simulink model "TST_AirCtl_DesValCalc"  (R2016b)
settings: Solver=FixedStepDiscrete  StartTime=0.0  StopTime=simTime  FixedStep=sampleTime  RelTol=1e-3
values from neighbouring files (symbols this model uses):
  testCase = 1    [initTST_AirCtl_DesValCalc_001.m]
libraries: simulink x4, UnitTest_Lib x2
settings Model: Creator=zhulinfeng  LastModifiedBy=zhulinfeng
settings DebuggingCC: SignalRangeChecking=error

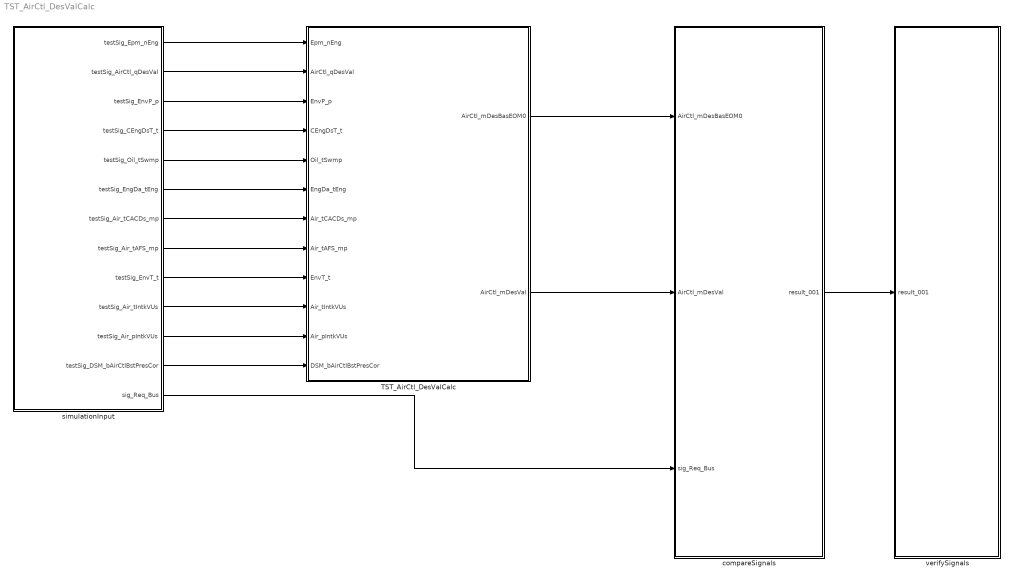
== system TST_AirCtl_DesValCalc ==
  TST_AirCtl_DesValCalc : Subsystem
  compareSignals : Subsystem
  simulationInput : Subsystem
  verifySignals : Subsystem
  wires:
  simulationInput/1(testSig_Epm_nEng) -> TST_AirCtl_DesValCalc/1(Epm_nEng)
  simulationInput/2(testSig_AirCtl_qDesVal) -> TST_AirCtl_DesValCalc/2(AirCtl_qDesVal)
  simulationInput/3(testSig_EnvP_p) -> TST_AirCtl_DesValCalc/3(EnvP_p)
  simulationInput/4(testSig_CEngDsT_t) -> TST_AirCtl_DesValCalc/4(CEngDsT_t)
  simulationInput/5(testSig_Oil_tSwmp) -> TST_AirCtl_DesValCalc/5(Oil_tSwmp)
  simulationInput/6(testSig_EngDa_tEng) -> TST_AirCtl_DesValCalc/6(EngDa_tEng)
  simulationInput/7(testSig_Air_tCACDs_mp) -> TST_AirCtl_DesValCalc/7(Air_tCACDs_mp)
  simulationInput/8(testSig_Air_tAFS_mp) -> TST_AirCtl_DesValCalc/8(Air_tAFS_mp)
  simulationInput/9(testSig_EnvT_t) -> TST_AirCtl_DesValCalc/9(EnvT_t)
  simulationInput/10(testSig_Air_tIntkVUs) -> TST_AirCtl_DesValCalc/10(Air_tIntkVUs)
  simulationInput/11(testSig_Air_pIntkVUs) -> TST_AirCtl_DesValCalc/11(Air_pIntkVUs)
  simulationInput/12(testSig_DSM_bAirCtlBstPresCor) -> TST_AirCtl_DesValCalc/12(DSM_bAirCtlBstPresCor)
  TST_AirCtl_DesValCalc/1(AirCtl_mDesBasEOM0) -> compareSignals/1(AirCtl_mDesBasEOM0)
  TST_AirCtl_DesValCalc/2(AirCtl_mDesVal) -> compareSignals/2(AirCtl_mDesVal)
  simulationInput/13(sig_Req_Bus) -> compareSignals/3(sig_Req_Bus)
  compareSignals/1(result_001) -> verifySignals/1(result_001)

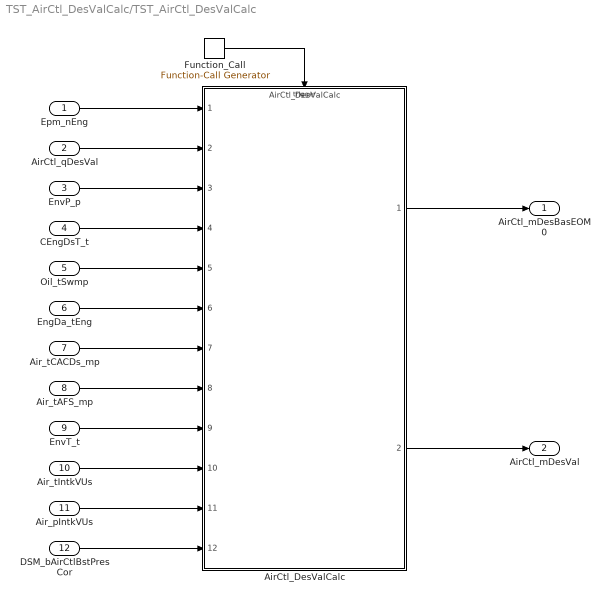
== system TST_AirCtl_DesValCalc/TST_AirCtl_DesValCalc ==
  Epm_nEng : Inport
  AirCtl_qDesVal : Inport  Port=2
  EnvP_p : Inport  Port=3
  CEngDsT_t : Inport  Port=4
  Oil_tSwmp : Inport  Port=5
  EngDa_tEng : Inport  Port=6
  Air_tCACDs_mp : Inport  Port=7
  Air_tAFS_mp : Inport  Port=8
  EnvT_t : Inport  Port=9
  Air_tIntkVUs : Inport  Port=10
  Air_pIntkVUs : Inport  Port=11
  DSM_bAirCtlBstPresCor : Inport  Port=12
  AirCtl_DesValCalc : ModelReference  ModelNameDialog=AirCtl_DesValCalc  SimulationMode=Normal  ModelReferenceVersion=1.18  TriggerPortName=function  TriggerPortTriggerType=function-call  TriggerPortStatesWhenEnabling=held
  Function_Call : simulink/Ports & Subsystems/Function-Call Generator  sample_time=sampleTime  numberOfIterations=1
  AirCtl_mDesBasEOM0 : Outport
  AirCtl_mDesVal : Outport  Port=2
  wires:
  Function_Call/1 -> AirCtl_DesValCalc/Trigger
  Epm_nEng/1 -> AirCtl_DesValCalc/1
  AirCtl_qDesVal/1 -> AirCtl_DesValCalc/2
  EnvP_p/1 -> AirCtl_DesValCalc/3
  CEngDsT_t/1 -> AirCtl_DesValCalc/4
  Oil_tSwmp/1 -> AirCtl_DesValCalc/5
  EngDa_tEng/1 -> AirCtl_DesValCalc/6
  Air_tCACDs_mp/1 -> AirCtl_DesValCalc/7
  Air_tAFS_mp/1 -> AirCtl_DesValCalc/8
  EnvT_t/1 -> AirCtl_DesValCalc/9
  Air_tIntkVUs/1 -> AirCtl_DesValCalc/10
  Air_pIntkVUs/1 -> AirCtl_DesValCalc/11
  DSM_bAirCtlBstPresCor/1 -> AirCtl_DesValCalc/12
  AirCtl_DesValCalc/1 -> AirCtl_mDesBasEOM0/1
  AirCtl_DesValCalc/2 -> AirCtl_mDesVal/1

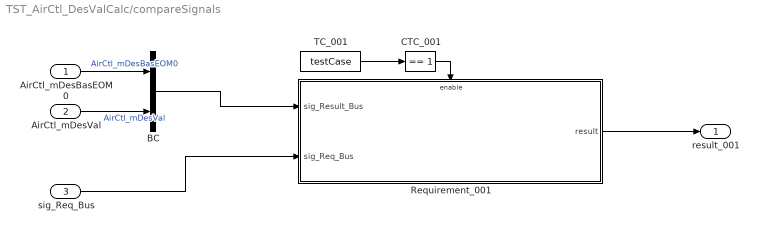
== system TST_AirCtl_DesValCalc/compareSignals ==
  AirCtl_mDesBasEOM0 : Inport
  AirCtl_mDesVal : Inport  Port=2
  sig_Req_Bus : Inport  Port=3
  BC : BusCreator  Inputs=2
  CTC_001 : simulink/Logic and Bit Operations/Compare To Constant  relop===  const=1  OutDataTypeStr=boolean
  Requirement_001 : Subsystem
  TC_001 : Constant  Value=testCase
  result_001 : Outport
  wires:
  AirCtl_mDesBasEOM0/1 -> BC/1  "AirCtl_mDesBasEOM0"
  AirCtl_mDesVal/1 -> BC/2  "AirCtl_mDesVal"
  TC_001/1 -> CTC_001/1
  CTC_001/1 -> Requirement_001/Enable
  sig_Req_Bus/1 -> Requirement_001/2(sig_Req_Bus)
  BC/1 -> Requirement_001/1(sig_Result_Bus)
  Requirement_001/1(result) -> result_001/1

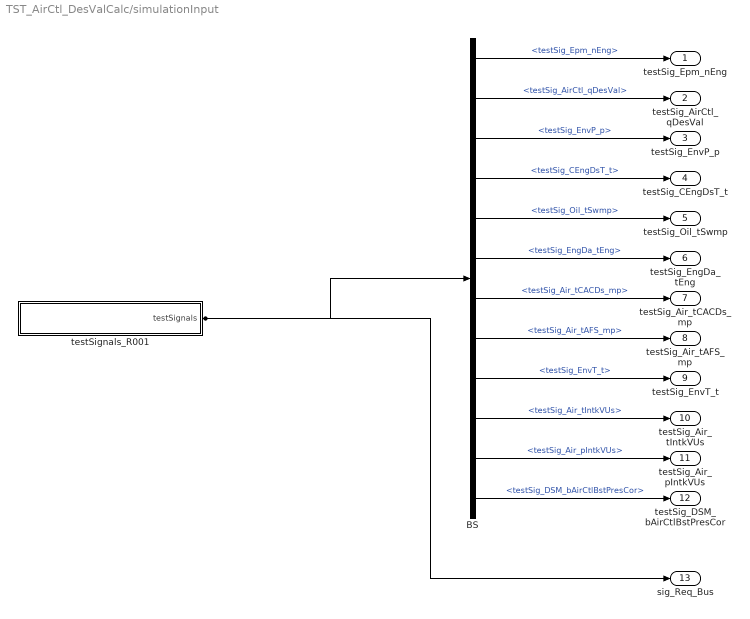
== system TST_AirCtl_DesValCalc/simulationInput ==
  BS : BusSelector  OutputSignals=testSig_Epm_nEng,testSig_AirCtl_qDesVal,testSig_EnvP_p,testSig_CEngDsT_t,testSig_Oil_tSwmp,testSig_EngDa_tEng,testSig_Air_tCACDs_mp,testSig_Air_tAFS_mp,testSig_EnvT_t,testSig_Air_tIntkVUs,testSig_Air_pIntkVUs,testSig_DSM_bAirCtlBstPresCor
  testSignals_R001 : Subsystem
  testSig_Epm_nEng : Outport
  testSig_AirCtl_qDesVal : Outport  Port=2
  testSig_EnvP_p : Outport  Port=3
  testSig_CEngDsT_t : Outport  Port=4
  testSig_Oil_tSwmp : Outport  Port=5
  testSig_EngDa_tEng : Outport  Port=6
  testSig_Air_tCACDs_mp : Outport  Port=7
  testSig_Air_tAFS_mp : Outport  Port=8
  testSig_EnvT_t : Outport  Port=9
  testSig_Air_tIntkVUs : Outport  Port=10
  testSig_Air_pIntkVUs : Outport  Port=11
  testSig_DSM_bAirCtlBstPresCor : Outport  Port=12
  sig_Req_Bus : Outport  Port=13
  wires:
  BS/1 -> testSig_Epm_nEng/1  "<testSig_Epm_nEng>"
  BS/2 -> testSig_AirCtl_qDesVal/1  "<testSig_AirCtl_qDesVal>"
  BS/3 -> testSig_EnvP_p/1  "<testSig_EnvP_p>"
  BS/4 -> testSig_CEngDsT_t/1  "<testSig_CEngDsT_t>"
  BS/5 -> testSig_Oil_tSwmp/1  "<testSig_Oil_tSwmp>"
  BS/6 -> testSig_EngDa_tEng/1  "<testSig_EngDa_tEng>"
  BS/7 -> testSig_Air_tCACDs_mp/1  "<testSig_Air_tCACDs_mp>"
  BS/8 -> testSig_Air_tAFS_mp/1  "<testSig_Air_tAFS_mp>"
  BS/9 -> testSig_EnvT_t/1  "<testSig_EnvT_t>"
  BS/10 -> testSig_Air_tIntkVUs/1  "<testSig_Air_tIntkVUs>"
  BS/11 -> testSig_Air_pIntkVUs/1  "<testSig_Air_pIntkVUs>"
  BS/12 -> testSig_DSM_bAirCtlBstPresCor/1  "<testSig_DSM_bAirCtlBstPresCor>"
  testSignals_R001/1(testSignals) -> BS/1, sig_Req_Bus/1

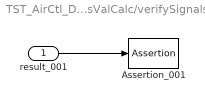
== system TST_AirCtl_DesValCalc/verifySignals ==
  result_001 : Inport
  Assertion_001 : Assertion  Enabled=off
  wires:
  result_001/1 -> Assertion_001/1

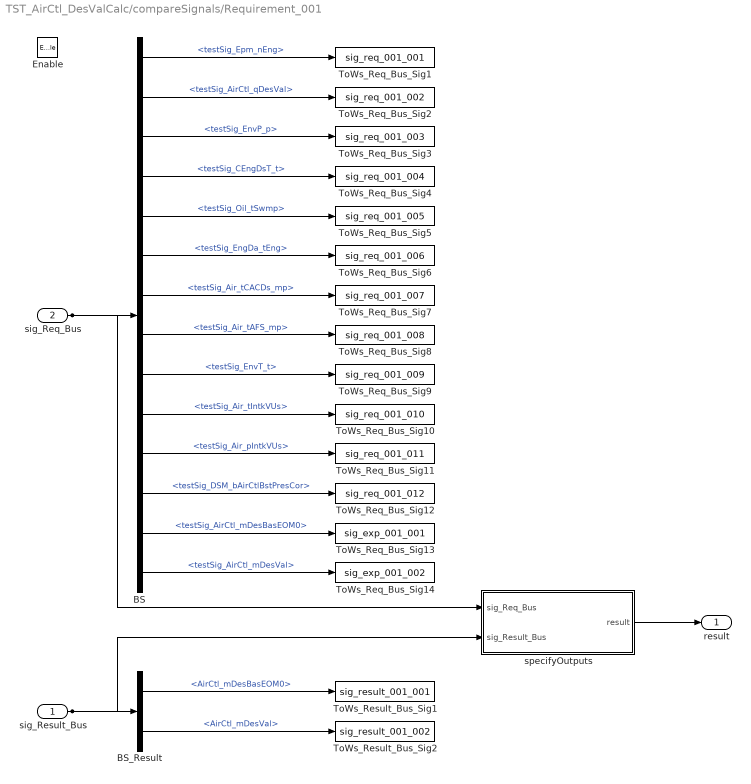
== system TST_AirCtl_DesValCalc/compareSignals/Requirement_001 ==
  sig_Result_Bus : Inport
  sig_Req_Bus : Inport  Port=2
  Enable : EnablePort
  BS : BusSelector  OutputSignals=testSig_Epm_nEng,testSig_AirCtl_qDesVal,testSig_EnvP_p,testSig_CEngDsT_t,testSig_Oil_tSwmp,testSig_EngDa_tEng,testSig_Air_tCACDs_mp,testSig_Air_tAFS_mp,testSig_EnvT_t,testSig_Air_tIntkVUs,testSig_Air_pIntkVUs,testSig_DSM_bAirCtlBstPresCor,testSig_AirCtl_mDesBasEOM0,testSig_AirCtl_mDesVal
  BS_Result : BusSelector  OutputSignals=AirCtl_mDesBasEOM0,AirCtl_mDesVal
  ToWs_Req_Bus_Sig1 : ToWorkspace  VariableName=sig_req_001_001  SaveFormat=Structure With Time
  ToWs_Req_Bus_Sig10 : ToWorkspace  VariableName=sig_req_001_010  SaveFormat=Structure With Time
  ToWs_Req_Bus_Sig11 : ToWorkspace  VariableName=sig_req_001_011  SaveFormat=Structure With Time
  ToWs_Req_Bus_Sig12 : ToWorkspace  VariableName=sig_req_001_012  SaveFormat=Structure With Time
  ToWs_Req_Bus_Sig13 : ToWorkspace  VariableName=sig_exp_001_001  SaveFormat=Structure With Time
  ToWs_Req_Bus_Sig14 : ToWorkspace  VariableName=sig_exp_001_002  SaveFormat=Structure With Time
  ToWs_Req_Bus_Sig2 : ToWorkspace  VariableName=sig_req_001_002  SaveFormat=Structure With Time
  ToWs_Req_Bus_Sig3 : ToWorkspace  VariableName=sig_req_001_003  SaveFormat=Structure With Time
  ToWs_Req_Bus_Sig4 : ToWorkspace  VariableName=sig_req_001_004  SaveFormat=Structure With Time
  ToWs_Req_Bus_Sig5 : ToWorkspace  VariableName=sig_req_001_005  SaveFormat=Structure With Time
  ToWs_Req_Bus_Sig6 : ToWorkspace  VariableName=sig_req_001_006  SaveFormat=Structure With Time
  ToWs_Req_Bus_Sig7 : ToWorkspace  VariableName=sig_req_001_007  SaveFormat=Structure With Time
  ToWs_Req_Bus_Sig8 : ToWorkspace  VariableName=sig_req_001_008  SaveFormat=Structure With Time
  ToWs_Req_Bus_Sig9 : ToWorkspace  VariableName=sig_req_001_009  SaveFormat=Structure With Time
  ToWs_Result_Bus_Sig1 : ToWorkspace  VariableName=sig_result_001_001  SaveFormat=Structure With Time
  ToWs_Result_Bus_Sig2 : ToWorkspace  VariableName=sig_result_001_002  SaveFormat=Structure With Time
  specifyOutputs : Subsystem
  result : Outport
  wires:
  sig_Req_Bus/1 -> BS/1, specifyOutputs/1(sig_Req_Bus)
  BS/1 -> ToWs_Req_Bus_Sig1/1  "<testSig_Epm_nEng>"
  BS/2 -> ToWs_Req_Bus_Sig2/1  "<testSig_AirCtl_qDesVal>"
  BS/3 -> ToWs_Req_Bus_Sig3/1  "<testSig_EnvP_p>"
  BS/4 -> ToWs_Req_Bus_Sig4/1  "<testSig_CEngDsT_t>"
  BS/5 -> ToWs_Req_Bus_Sig5/1  "<testSig_Oil_tSwmp>"
  BS/6 -> ToWs_Req_Bus_Sig6/1  "<testSig_EngDa_tEng>"
  BS/7 -> ToWs_Req_Bus_Sig7/1  "<testSig_Air_tCACDs_mp>"
  BS/8 -> ToWs_Req_Bus_Sig8/1  "<testSig_Air_tAFS_mp>"
  BS/9 -> ToWs_Req_Bus_Sig9/1  "<testSig_EnvT_t>"
  BS/10 -> ToWs_Req_Bus_Sig10/1  "<testSig_Air_tIntkVUs>"
  BS/11 -> ToWs_Req_Bus_Sig11/1  "<testSig_Air_pIntkVUs>"
  BS/12 -> ToWs_Req_Bus_Sig12/1  "<testSig_DSM_bAirCtlBstPresCor>"
  BS/13 -> ToWs_Req_Bus_Sig13/1  "<testSig_AirCtl_mDesBasEOM0>"
  BS/14 -> ToWs_Req_Bus_Sig14/1  "<testSig_AirCtl_mDesVal>"
  sig_Result_Bus/1 -> BS_Result/1, specifyOutputs/2(sig_Result_Bus)
  BS_Result/1 -> ToWs_Result_Bus_Sig1/1  "<AirCtl_mDesBasEOM0>"
  BS_Result/2 -> ToWs_Result_Bus_Sig2/1  "<AirCtl_mDesVal>"
  specifyOutputs/1(result) -> result/1

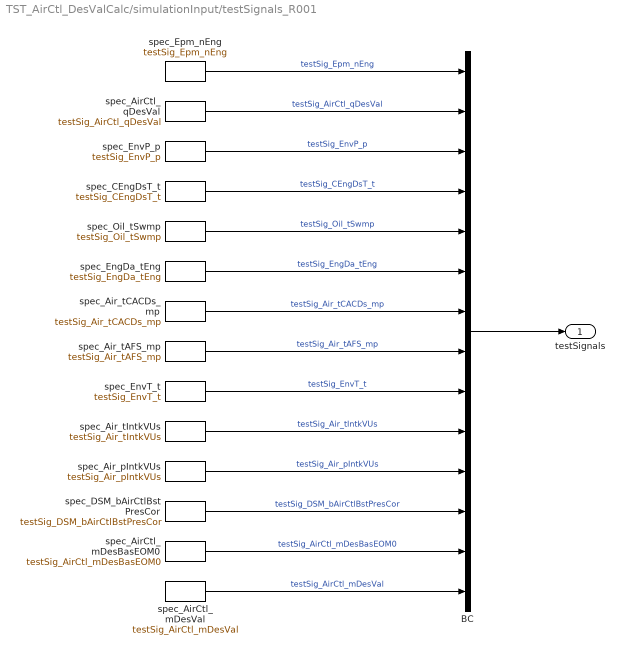
== system TST_AirCtl_DesValCalc/simulationInput/testSignals_R001 ==
  BC : BusCreator  Inputs=14
  spec_AirCtl_mDesBasEOM0 : FromWorkspace  VariableName=testSig_AirCtl_mDesBasEOM0  Interpolate=off  OutputAfterFinalValue=Holding final value
  spec_AirCtl_mDesVal : FromWorkspace  VariableName=testSig_AirCtl_mDesVal  Interpolate=off  OutputAfterFinalValue=Holding final value
  spec_AirCtl_qDesVal : FromWorkspace  VariableName=testSig_AirCtl_qDesVal  Interpolate=off  OutputAfterFinalValue=Holding final value
  spec_Air_pIntkVUs : FromWorkspace  VariableName=testSig_Air_pIntkVUs  Interpolate=off  OutputAfterFinalValue=Holding final value
  spec_Air_tAFS_mp : FromWorkspace  VariableName=testSig_Air_tAFS_mp  Interpolate=off  OutputAfterFinalValue=Holding final value
  spec_Air_tCACDs_mp : FromWorkspace  VariableName=testSig_Air_tCACDs_mp  Interpolate=off  OutputAfterFinalValue=Holding final value
  spec_Air_tIntkVUs : FromWorkspace  VariableName=testSig_Air_tIntkVUs  Interpolate=off  OutputAfterFinalValue=Holding final value
  spec_CEngDsT_t : FromWorkspace  VariableName=testSig_CEngDsT_t  Interpolate=off  OutputAfterFinalValue=Holding final value
  spec_DSM_bAirCtlBstPresCor : FromWorkspace  VariableName=testSig_DSM_bAirCtlBstPresCor  Interpolate=off  OutputAfterFinalValue=Holding final value
  spec_EngDa_tEng : FromWorkspace  VariableName=testSig_EngDa_tEng  Interpolate=off  OutputAfterFinalValue=Holding final value
  spec_EnvP_p : FromWorkspace  VariableName=testSig_EnvP_p  Interpolate=off  OutputAfterFinalValue=Holding final value
  spec_EnvT_t : FromWorkspace  VariableName=testSig_EnvT_t  Interpolate=off  OutputAfterFinalValue=Holding final value
  spec_Epm_nEng : FromWorkspace  VariableName=testSig_Epm_nEng  Interpolate=off  OutputAfterFinalValue=Holding final value
  spec_Oil_tSwmp : FromWorkspace  VariableName=testSig_Oil_tSwmp  Interpolate=off  OutputAfterFinalValue=Holding final value
  testSignals : Outport
  wires:
  BC/1 -> testSignals/1
  spec_Epm_nEng/1 -> BC/1  "testSig_Epm_nEng"
  spec_AirCtl_qDesVal/1 -> BC/2  "testSig_AirCtl_qDesVal"
  spec_EnvP_p/1 -> BC/3  "testSig_EnvP_p"
  spec_CEngDsT_t/1 -> BC/4  "testSig_CEngDsT_t"
  spec_Oil_tSwmp/1 -> BC/5  "testSig_Oil_tSwmp"
  spec_EngDa_tEng/1 -> BC/6  "testSig_EngDa_tEng"
  spec_Air_tCACDs_mp/1 -> BC/7  "testSig_Air_tCACDs_mp"
  spec_Air_tAFS_mp/1 -> BC/8  "testSig_Air_tAFS_mp"
  spec_EnvT_t/1 -> BC/9  "testSig_EnvT_t"
  spec_Air_tIntkVUs/1 -> BC/10  "testSig_Air_tIntkVUs"
  spec_Air_pIntkVUs/1 -> BC/11  "testSig_Air_pIntkVUs"
  spec_DSM_bAirCtlBstPresCor/1 -> BC/12  "testSig_DSM_bAirCtlBstPresCor"
  spec_AirCtl_mDesBasEOM0/1 -> BC/13  "testSig_AirCtl_mDesBasEOM0"
  spec_AirCtl_mDesVal/1 -> BC/14  "testSig_AirCtl_mDesVal"

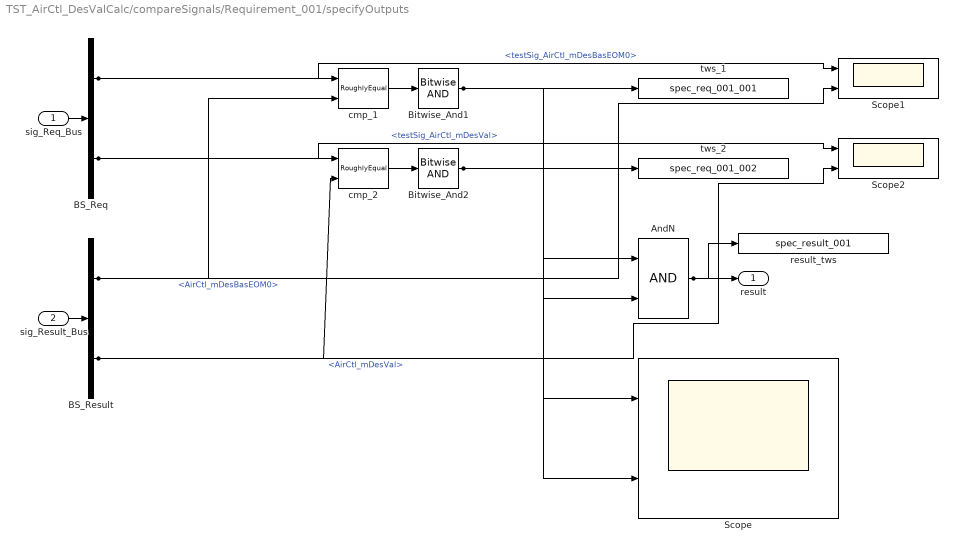
== system TST_AirCtl_DesValCalc/compareSignals/Requirement_001/specifyOutputs ==
  sig_Req_Bus : Inport
  sig_Result_Bus : Inport  Port=2
  AndN : Logic
  BS_Req : BusSelector  OutputSignals=testSig_AirCtl_mDesBasEOM0,testSig_AirCtl_mDesVal
  BS_Result : BusSelector  OutputSignals=AirCtl_mDesBasEOM0,AirCtl_mDesVal
  Bitwise_And1 : simulink/Logic and Bit Operations/Bitwise Operator  logicop=AND  UseBitMask=off  BitMask=bin2dec('11011001')  BitMaskRealWorld=Stored Integer
  Bitwise_And2 : simulink/Logic and Bit Operations/Bitwise Operator  logicop=AND  UseBitMask=off  BitMask=bin2dec('11011001')  BitMaskRealWorld=Stored Integer
  Scope : Scope  NumInputPorts=2
  Scope1 : Scope  NumInputPorts=2
  Scope2 : Scope  NumInputPorts=2
  cmp_1 : UnitTest_Lib/RoughlyEqual  slope=0.1
  cmp_2 : UnitTest_Lib/RoughlyEqual  slope=0.1
  result_tws : ToWorkspace  VariableName=spec_result_001
  tws_1 : ToWorkspace  VariableName=spec_req_001_001
  tws_2 : ToWorkspace  VariableName=spec_req_001_002
  result : Outport
  wires:
  sig_Req_Bus/1 -> BS_Req/1
  sig_Result_Bus/1 -> BS_Result/1
  AndN/1 -> result/1, result_tws/1
  BS_Req/1 -> cmp_1/1, Scope1/1  "<testSig_AirCtl_mDesBasEOM0>"
  BS_Result/1 -> cmp_1/2, Scope1/2  "<AirCtl_mDesBasEOM0>"
  cmp_1/1 -> Bitwise_And1/1
  Bitwise_And1/1 -> tws_1/1, AndN/1, Scope/1
  BS_Req/2 -> cmp_2/1, Scope2/1  "<testSig_AirCtl_mDesVal>"
  BS_Result/2 -> cmp_2/2, Scope2/2  "<AirCtl_mDesVal>"
  cmp_2/1 -> Bitwise_And2/1
  Bitwise_And2/1 -> tws_2/1, AndN/2, Scope/2
